simulink model "simulation_adaptatif_idp"  (R2020a)
settings: Solver=VariableStepAuto  StartTime=0.0  StopTime=10  RelTol=1e-3
values from neighbouring files (symbols this model uses):
  a = 1    [Adap.m]    (also in Adaptive_control_Non_linear.m = 2; HOSM.m; projet_AAV.m; sys.m)
  b = 2    [Adaptive_Control_Linear.m]    (also in Adaptive_control_Non_linear.m; HOSM.m = 1; feedback-integrator.m = 3; mini_projet.m = 3)
  gamma1 = 0.5    [Adaptive_Control_Linear.m]    (also in Adaptive_control_Non_linear.m; projet_AAV.m = 1000)
  gamma2 = 0.5    [Adaptive_Control_Linear.m]    (also in Adaptive_control_Non_linear.m; projet_AAV.m = 1000)
  lambda = 0.3    [fuzzy.m]    (also in projet_AAV.m = 1)
settings Model: Creator=amine  LastModifiedBy=lenovo

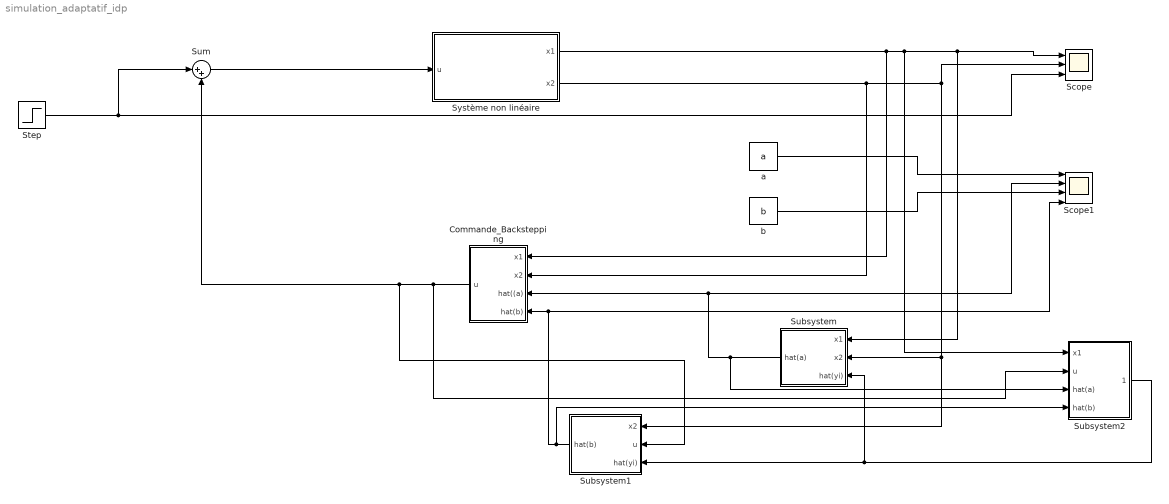
== system simulation_adaptatif_idp ==
  Commande_Backstepping : Subsystem
  Scope : Scope  NumInputPorts=3
  Scope1 : Scope  NumInputPorts=4
  Step : Step  Time=0  SampleTime=0
  Subsystem : Subsystem
  Subsystem1 : Subsystem
  Subsystem2 : Subsystem
  Sum : Sum  Inputs=|++
  Système non linéaire : Subsystem
  a : Constant  Value=a  OutDataTypeStr=Inherit: Inherit via back propagation
  b : Constant  Value=b  OutDataTypeStr=Inherit: Inherit via back propagation
  wires:
  a/1 -> Scope1/1
  Commande_Backstepping/1(u) -> Subsystem2/2(u), Subsystem1/2(u), Sum/2
  Step/1 -> Scope/3, Sum/1
  Subsystem/1(hat(a)) -> Scope1/2, Commande_Backstepping/3(hat((a)), Subsystem2/3(hat(a))
  Sum/1 -> Système non linéaire/1(u)
  Système non linéaire/2(x2) -> Scope/2, Subsystem1/1(x2), Subsystem/2(x2), Commande_Backstepping/2(x2)
  Subsystem1/1(hat(b)) -> Subsystem2/4(hat(b)), Commande_Backstepping/4(hat(b)), Scope1/4
  Système non linéaire/1(x1) -> Subsystem2/1(x1), Scope/1, Subsystem/1(x1), Commande_Backstepping/1(x1)
  Subsystem2/1(hat(yi)) -> Subsystem1/3(hat(yi)), Subsystem/3(hat(yi))
  b/1 -> Scope1/3

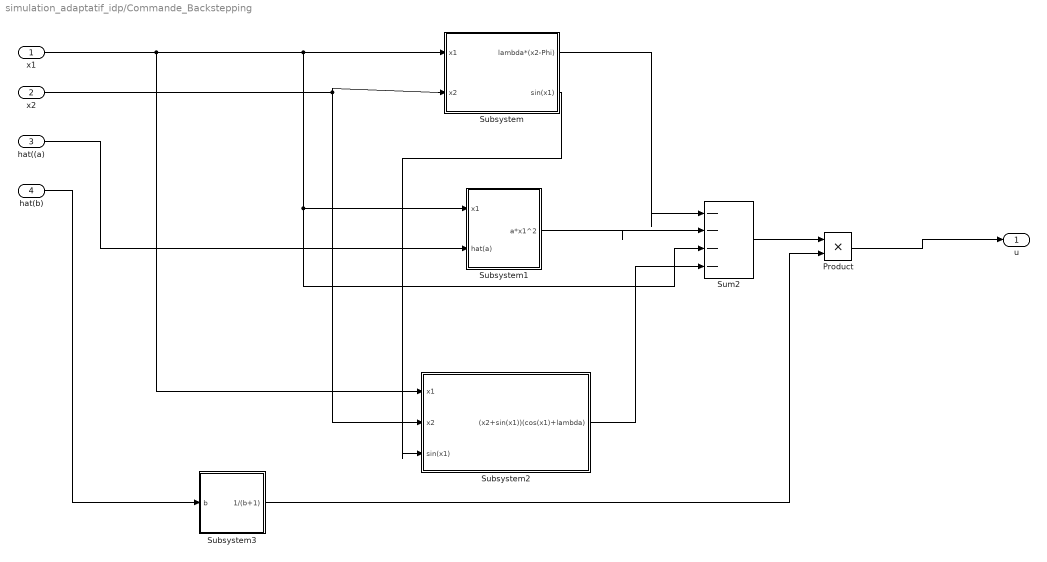
== system simulation_adaptatif_idp/Commande_Backstepping ==
  x1 : Inport
  x2 : Inport  Port=2
  hat((a) : Inport  Port=3
  hat(b) : Inport  Port=4
  Product : Product
  Subsystem : Subsystem
  Subsystem1 : Subsystem
  Subsystem2 : Subsystem
  Subsystem3 : Subsystem
  Sum2 : Sum  Inputs=|----
  u : Outport
  wires:
  x1/1 -> Subsystem2/1("x1 "), Subsystem/1(x1), Sum2/3, Subsystem1/1("x1 ")
  x2/1 -> Subsystem2/2(x2), Subsystem/2(x2)
  Sum2/1 -> Product/1
  Product/1 -> u/1
  Subsystem/1(lambda*(x2-Phi)) -> Sum2/1
  Subsystem1/1(a*x1^2) -> Sum2/2
  Subsystem/2(sin(x1)) -> Subsystem2/3(sin(x1))
  Subsystem2/1((x2+sin(x1))(cos(x1)+lambda)) -> Sum2/4
  hat((a)/1 -> Subsystem1/2(hat(a))
  hat(b)/1 -> Subsystem3/1(b)
  Subsystem3/1(1/(b+1)) -> Product/2

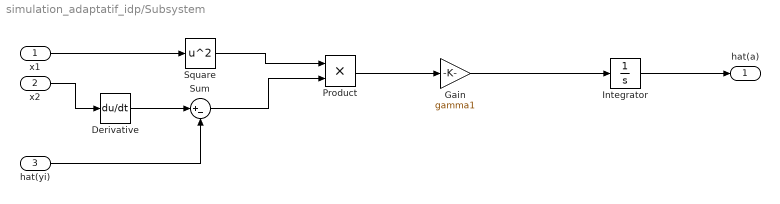
== system simulation_adaptatif_idp/Subsystem ==
  x1 : Inport
  x2 : Inport  Port=2
  hat(yi) : Inport  Port=3
  Derivative : Derivative
  Gain : Gain  Gain=gamma1
  Integrator : Integrator  LimitOutput=on  UpperSaturationLimit=1  LowerSaturationLimit=-1
  Product : Product
  Square : Math  Operator=square  SaturateOnIntegerOverflow=on
  Sum : Sum  Inputs=|+-
  hat(a) : Outport
  wires:
  Gain/1 -> Integrator/1
  x2/1 -> Derivative/1
  Derivative/1 -> Sum/1
  hat(yi)/1 -> Sum/2
  x1/1 -> Square/1
  Square/1 -> Product/1
  Sum/1 -> Product/2
  Product/1 -> Gain/1
  Integrator/1 -> hat(a)/1

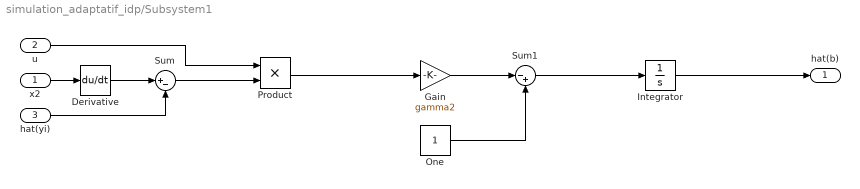
== system simulation_adaptatif_idp/Subsystem1 ==
  x2 : Inport
  u : Inport  Port=2
  hat(yi) : Inport  Port=3
  Derivative : Derivative
  Gain : Gain  Gain=gamma2
  Integrator : Integrator  InitialCondition=-0.25  LimitOutput=on  UpperSaturationLimit=0.25  LowerSaturationLimit=-0.25
  One : Constant  OutDataTypeStr=Inherit: Inherit via back propagation
  Product : Product
  Sum : Sum  Inputs=|+-
  Sum1 : Sum  Inputs=|-+
  hat(b) : Outport
  wires:
  x2/1 -> Derivative/1
  Derivative/1 -> Sum/1
  hat(yi)/1 -> Sum/2
  Sum/1 -> Product/2
  u/1 -> Product/1
  Product/1 -> Gain/1
  Gain/1 -> Sum1/1
  One/1 -> Sum1/2
  Sum1/1 -> Integrator/1
  Integrator/1 -> hat(b)/1

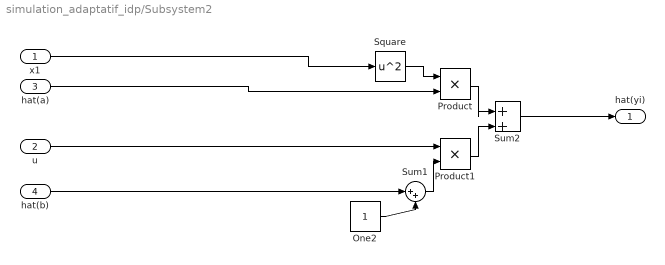
== system simulation_adaptatif_idp/Subsystem2 ==
  x1 : Inport
  u : Inport  Port=2
  hat(a) : Inport  Port=3
  hat(b) : Inport  Port=4
  One2 : Constant  OutDataTypeStr=Inherit: Inherit via back propagation
  Product : Product
  Product1 : Product
  Square : Math  Operator=square  SaturateOnIntegerOverflow=on
  Sum1 : Sum  Inputs=|++
  Sum2 : Sum  Inputs=|++
  hat(yi) : Outport
  wires:
  Square/1 -> Product/1
  Sum1/1 -> Product1/2
  x1/1 -> Square/1
  One2/1 -> Sum1/2
  Product1/1 -> Sum2/2
  Product/1 -> Sum2/1
  hat(b)/1 -> Sum1/1
  Sum2/1 -> hat(yi)/1
  u/1 -> Product1/1
  hat(a)/1 -> Product/2

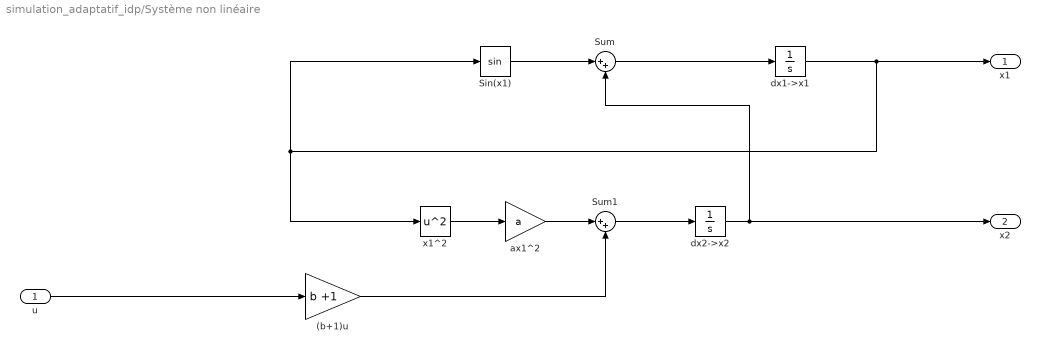
== system simulation_adaptatif_idp/Système non linéaire ==
  u : Inport
  (b+1)u : Gain  Gain=b +1
  Sin(x1) : Trigonometry
  Sum : Sum  Inputs=|++
  Sum1 : Sum  Inputs=|++
  ax1^2 : Gain  Gain=a
  dx1->x1 : Integrator
  dx2->x2 : Integrator
  x1^2 : Math  Operator=square  SaturateOnIntegerOverflow=on
  x1 : Outport
  x2 : Outport  Port=2
  wires:
  (b+1)u/1 -> Sum1/2
  dx2->x2/1 -> x2/1, Sum/2
  u/1 -> (b+1)u/1
  ax1^2/1 -> Sum1/1
  dx1->x1/1 -> Sin(x1)/1, x1^2/1, x1/1
  Sin(x1)/1 -> Sum/1
  x1^2/1 -> ax1^2/1
  Sum1/1 -> dx2->x2/1
  Sum/1 -> dx1->x1/1

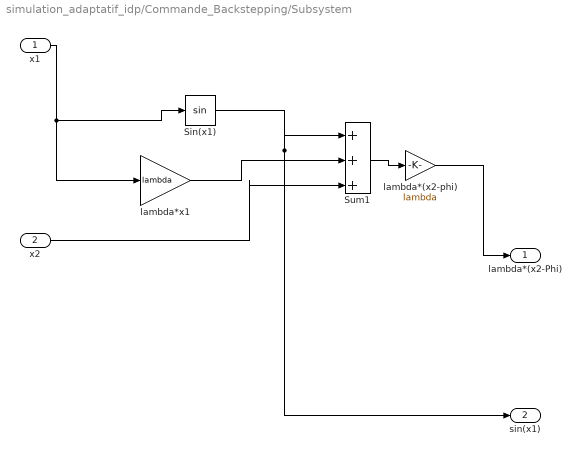
== system simulation_adaptatif_idp/Commande_Backstepping/Subsystem ==
  x1 : Inport
  x2 : Inport  Port=2
  Sin(x1) : Trigonometry
  Sum1 : Sum  Inputs=|+++
  lambda*(x2-phi) : Gain  Gain=lambda
  lambda*x1 : Gain  Gain=lambda
  lambda*(x2-Phi) : Outport
  sin(x1) : Outport  Port=2
  wires:
  x1/1 -> Sin(x1)/1, lambda*x1/1
  Sin(x1)/1 -> sin(x1)/1, Sum1/1
  Sum1/1 -> lambda*(x2-phi)/1
  x2/1 -> Sum1/3
  lambda*x1/1 -> Sum1/2
  lambda*(x2-phi)/1 -> lambda*(x2-Phi)/1

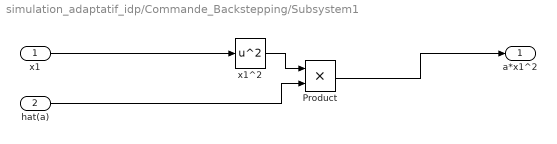
== system simulation_adaptatif_idp/Commande_Backstepping/Subsystem1 ==
  "x1 " : Inport
  hat(a) : Inport  Port=2
  Product : Product
  x1^2 : Math  Operator=square  SaturateOnIntegerOverflow=on
  a*x1^2 : Outport
  wires:
  x1^2/1 -> Product/1
  Product/1 -> a*x1^2/1
  "x1 "/1 -> x1^2/1
  hat(a)/1 -> Product/2

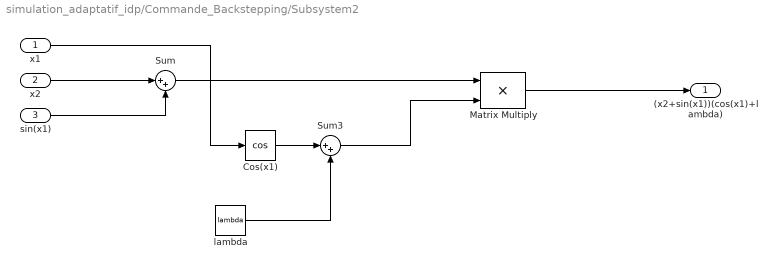
== system simulation_adaptatif_idp/Commande_Backstepping/Subsystem2 ==
  "x1 " : Inport
  x2 : Inport  Port=2
  sin(x1) : Inport  Port=3
  Cos(x1) : Trigonometry  Operator=cos
  Matrix Multiply : Product
  Sum : Sum  Inputs=|++
  Sum3 : Sum  Inputs=|++
  lambda : Constant  Value=lambda  OutDataTypeStr=Inherit: Inherit via back propagation
  (x2+sin(x1))(cos(x1)+lambda) : Outport
  wires:
  Cos(x1)/1 -> Sum3/1
  sin(x1)/1 -> Sum/2
  lambda/1 -> Sum3/2
  x2/1 -> Sum/1
  Matrix Multiply/1 -> (x2+sin(x1))(cos(x1)+lambda)/1
  Sum/1 -> Matrix Multiply/1
  Sum3/1 -> Matrix Multiply/2
  "x1 "/1 -> Cos(x1)/1

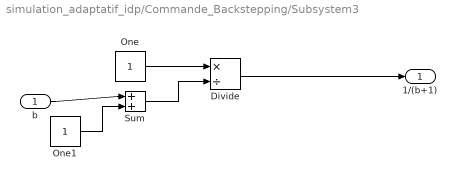
== system simulation_adaptatif_idp/Commande_Backstepping/Subsystem3 ==
  b : Inport
  Divide : Product  Inputs=*/
  One : Constant  OutDataTypeStr=Inherit: Inherit via back propagation
  One1 : Constant  OutDataTypeStr=Inherit: Inherit via back propagation
  Sum : Sum  Inputs=|++
  1/(b+1) : Outport
  wires:
  Sum/1 -> Divide/2
  One/1 -> Divide/1
  One1/1 -> Sum/2
  b/1 -> Sum/1
  Divide/1 -> 1/(b+1)/1
